simulink model "Subsystem2"  (R2020b)
settings: Solver=FixedStepAuto  StartTime=0.0  StopTime=10.0  FixedStep=1  MaxStep=1  RelTol=1e-3
model workspace (MAT data in the model file):
  K11 = 1
  K12 = 2
  K13 = -1
  K21 = 1
  K22 = 1
  K23 = -1
settings Model: DataDictionary=Data.sldd  Creator=user  LastModifiedBy=user
settings DataIOCC: SaveOutput=off  SaveTime=off

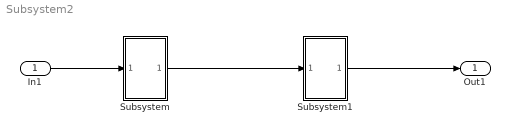
== system Subsystem2 ==
  In1 : Inport  OutDataTypeStr=double  PortDimensions=1  SampleTime=0
  Subsystem : Subsystem
  Subsystem1 : Subsystem
  Out1 : Outport  OutDataTypeStr=double  PortDimensions=1  SampleTime=0
  wires:
  Subsystem/1(Out1) -> Subsystem1/1(In1)
  In1/1 -> Subsystem/1(In1)
  Subsystem1/1(Out1) -> Out1/1

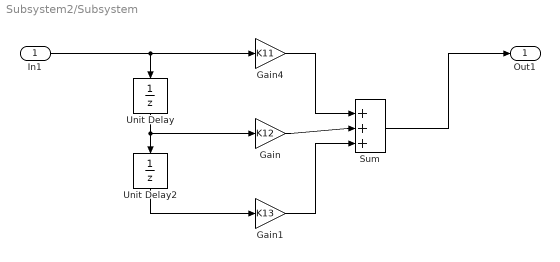
== system Subsystem2/Subsystem ==
  In1 : Inport
  Gain : Gain  Gain=K12
  Gain1 : Gain  Gain=K13
  Gain4 : Gain  Gain=K11
  Sum : Sum  Inputs=+|++
  Unit Delay : UnitDelay  SampleTime=-1  HasFrameUpgradeWarning=on
  Unit Delay2 : UnitDelay  SampleTime=-1  HasFrameUpgradeWarning=on
  Out1 : Outport
  wires:
  Sum/1 -> Out1/1
  Gain/1 -> Sum/2
  Gain1/1 -> Sum/3
  Unit Delay2/1 -> Gain1/1
  In1/1 -> Unit Delay/1, Gain4/1
  Unit Delay/1 -> Gain/1, Unit Delay2/1
  Gain4/1 -> Sum/1

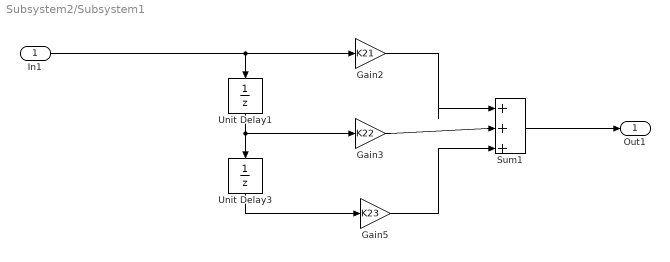
== system Subsystem2/Subsystem1 ==
  In1 : Inport
  Gain2 : Gain  Gain=K21
  Gain3 : Gain  Gain=K22
  Gain5 : Gain  Gain=K23
  Sum1 : Sum  Inputs=|+++
  Unit Delay1 : UnitDelay  SampleTime=-1  HasFrameUpgradeWarning=on
  Unit Delay3 : UnitDelay  SampleTime=-1  HasFrameUpgradeWarning=on
  Out1 : Outport
  wires:
  Gain3/1 -> Sum1/2
  Unit Delay3/1 -> Gain5/1
  In1/1 -> Gain2/1, Unit Delay1/1
  Gain5/1 -> Sum1/3
  Sum1/1 -> Out1/1
  Unit Delay1/1 -> Unit Delay3/1, Gain3/1
  Gain2/1 -> Sum1/1
